simulink model "ploopControl"  (R2023b)
settings: Solver=ode15s  StartTime=0.0  StopTime=1  RelTol=1e-3  EnableMultiTasking=on
undefined symbols (not defined in the file or in its folder): G
libraries: roblocks x2
settings Model: Creator=pic  LastModifiedBy=dell
settings SolverCC: AlgebraicLoopSolver=TrustRegion
settings DataIOCC: SaveFormat=Array  SignalLoggingSaveFormat=ModelDataLogs  TimeSaveName=t  OutputSaveName=y  OutputOption=SpecifiedOutputTimes  OutputTimes=[0:0.001:1]'
settings OptimizationCC: ExpressionDepthLimit=2147483647  LifeSpan=inf
settings DebuggingCC: UnderspecifiedInitializationDetection=Classic  MergeDetectMultiDrivingBlocksExec=none  SolverPrmCheckMsg=warning  UnconnectedInputMsg=warning  UnconnectedOutputMsg=warning  UnconnectedLineMsg=warning  AllowSymbolicDim=off  StateNameClashWarn=warning  SFUnexpectedBacktrackingDiag=warning  SFNoUnconditionalDefaultTransitionDiag=warning  SFExecutionAtInitializationDiag=none  ArithmeticOperatorsInVariantConditions=warning
settings HardwareCC: ProdBitPerPointer=32  ProdBitPerSizeT=32  ProdBitPerPtrDiffT=32  ProdLargestAtomicFloat=None  ProdIntDivRoundTo=Undefined  ProdEndianess=Unspecified  ProdWordSize=32  ProdHWDeviceType=32-bit Generic
settings ModelReferenceCC: EnableRefExpFcnMdlSchedulingChecks=on  PropagateSignalLabelsOutOfModel=off
settings SFSimCC: SimUseLocalCustomCode=off  CustomCodeUndefinedFunction=UseInterfaceOnly
settings RTWCC: RTWUseLocalCustomCode=off
settings CodeAppCC: StateflowObjectComments=on
settings GRTTargetCC: TargetLangStandard=C89/C90 (ANSI)  CombineOutputUpdateFcns=off  GRTInterface=on
settings ConfigComp: CovMetricSettings=dw  CovSaveCumulativeToWorkspaceVar=on  CovSaveSingleToWorkspaceVar=on  CovExternalEMLEnable=off  CovSFcnEnable=off

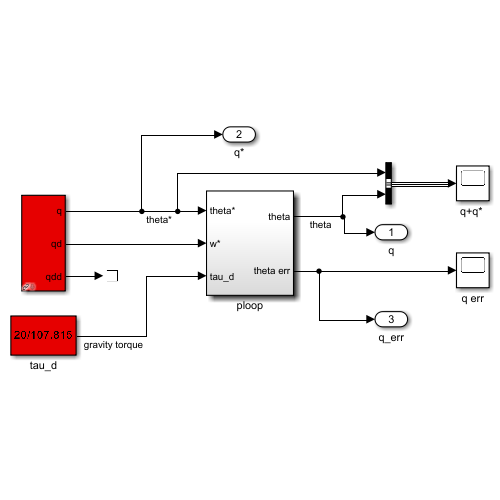
[thumbnail: Simulink's stored preview of the top-level diagram]
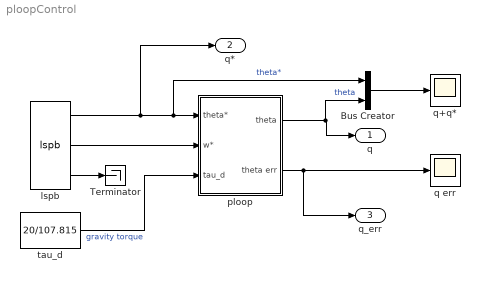
== system ploopControl ==
  Bus Creator : BusCreator  Inputs=2
  Terminator : Terminator
  lspb : roblocks/Toolbox/lspb  q0=0  qf=1  tmax=1
  ploop : Subsystem
  q err : Scope
  "q+q* " : Scope
  tau_d : Constant  Value=20/107.815
  q : Outport  VectorParamsAs1DForOutWhenUnconnected=off
  q* : Outport  Port=2  VectorParamsAs1DForOutWhenUnconnected=off
  q_err : Outport  Port=3  VectorParamsAs1DForOutWhenUnconnected=off
  wires:
  ploop/1(theta) -> Bus Creator/2, q/1  "theta"
  ploop/2(theta err) -> q_err/1, q err/1
  lspb/1 -> q*/1, Bus Creator/1, ploop/1(theta*)  "theta*"
  tau_d/1 -> ploop/3(tau_d)  "gravity torque"
  lspb/3 -> Terminator/1
  lspb/2 -> ploop/2(w*)
  Bus Creator/1 -> "q+q* "/1

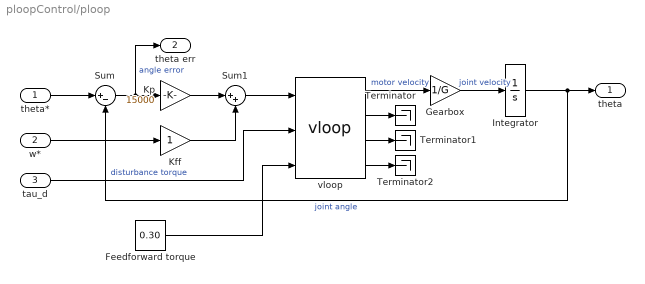
== system ploopControl/ploop ==
  theta* : Inport
  w* : Inport  Port=2
  tau_d : Inport  Port=3
  Feedforward torque : Constant  Value=0.30
  Gearbox : Gain  Gain=1/G
  Integrator : Integrator
  Kff : Gain
  Kp : Gain  Gain=15000
  Sum : Sum  Inputs=|+-
  Sum1 : Sum  Inputs=|++
  Terminator : Terminator
  Terminator1 : Terminator
  Terminator2 : Terminator
  vloop : roblocks/Arm/vloop  J=372e-6  B=817e-6  Km=0.228  tau_max=0.9  Kv=1  Ki=10  T=0.001
  theta : Outport  VectorParamsAs1DForOutWhenUnconnected=off
  theta err : Outport  Port=2  VectorParamsAs1DForOutWhenUnconnected=off
  wires:
  Sum/1 -> Kp/1, theta err/1  "angle error"
  Integrator/1 -> theta/1, Sum/2  "joint angle"
  theta*/1 -> Sum/1
  Kp/1 -> Sum1/1
  Sum1/1 -> vloop/1
  w*/1 -> Kff/1
  Kff/1 -> Sum1/2
  vloop/2 -> Terminator/1
  vloop/3 -> Terminator1/1
  vloop/4 -> Terminator2/1
  vloop/1 -> Gearbox/1  "motor velocity"
  tau_d/1 -> vloop/2  "disturbance torque"
  Feedforward torque/1 -> vloop/3
  Gearbox/1 -> Integrator/1  "joint velocity"
